simulink model "KalmanfilterReal"  (R2015a)
settings: Solver=ode3  StartTime=0.0  StopTime=10.0  FixedStep=1/200  RelTol=1e-3
undefined symbols (not defined in the file or in its folder): i
libraries: PoliArd x6
settings Model: ExtModeTrigDuration=2  Creator=User  LastModifiedBy=user
settings OptimizationCC: OptimizeModelRefInitCode=on  LifeSpan=1
settings DebuggingCC: UnderspecifiedInitializationDetection=Classic  MergeDetectMultiDrivingBlocksExec=none
settings HardwareCC: ProdLargestAtomicInteger=Long  ProdLargestAtomicFloat=Double  ProdEndianess=LittleEndian  ProdHWDeviceType=ARM Compatible->ARM Cortex
settings RTWCC: SystemTargetFile=realtime.tlc  GenerateMakefile=off  TemplateMakefile=realtime.tmf  Description=Run on Target Hardware  RTWVerbose=off
settings ERTTargetCC: CombineOutputUpdateFcns=off  ExtModeTransport=3  ExtModeMexFile=ext_serial_win32_comm_rtt  ExtModeMexArgs=0 1 9600  ERTSrcFileBannerTemplate=realtime_code_template.cgt  ERTHdrFileBannerTemplate=realtime_code_template.cgt  ERTDataSrcFileTemplate=realtime_code_template.cgt  ERTDataHdrFileTemplate=realtime_code_template.cgt  ERTCustomFileTemplate=realtime_file_process.tlc

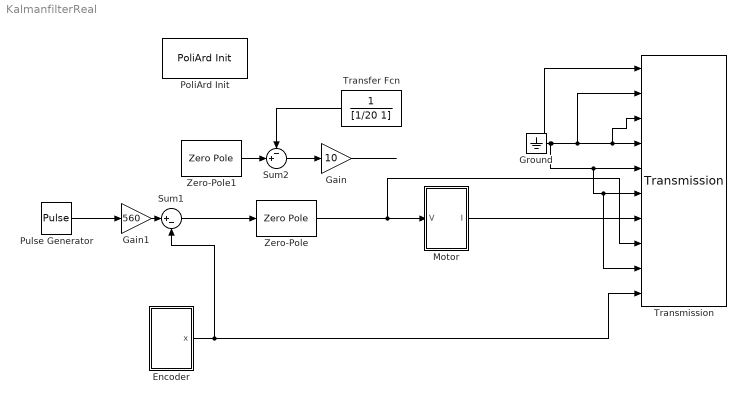
== system KalmanfilterReal ==
  "Encoder " : Subsystem
  Gain : Gain  Gain=10
  Gain1 : Gain  Gain=560
  Ground : Ground
  Motor : Subsystem
  PoliArd Init : PoliArd/PoliArd Init
  Pulse Generator : DiscretePulseGenerator  PulseType=Time based  Amplitude=-2.5  Period=10  PulseWidth=50  PhaseDelay=500
  Sum1 : Sum  Inputs=|+-
  Sum2 : Sum  Inputs=-+|
  Transfer Fcn : TransferFcn  Denominator=[1/20 1]
  Transmission : PoliArd/Transmission  sample_freq=200  sig_to_send=6
  Zero-Pole : ZeroPole  Zeros=[3.0405+i*12.6,3.0405-i*12.6]  Poles=[0 -200]  Gain=[-0.038702]
  Zero-Pole1 : ZeroPole  Zeros=[-2+22i, -2-22i]  Poles=[0, -100]  Gain=-0.1
  wires:
  Motor/1(I) -> Transmission/7
  Ground/1 -> Transmission/1, Transmission/9, Transmission/6, Transmission/5, Transmission/2, Transmission/3, Transmission/4
  Gain/1 -> ?
  Sum2/1 -> Gain/1
  Zero-Pole1/1 -> Sum2/2
  Transfer Fcn/1 -> Sum2/1
  Sum1/1 -> Zero-Pole/1
  Gain1/1 -> Sum1/1
  "Encoder "/1(x) -> Transmission/10, Sum1/2
  Zero-Pole/1 -> Transmission/8, Motor/1(V)
  Pulse Generator/1 -> Gain1/1

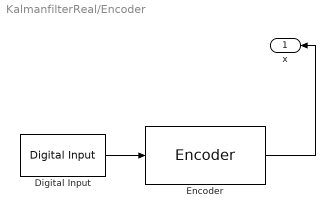
== system KalmanfilterReal/Encoder  ==
  Digital Input : PoliArd/Digital Input  DI_pin=2  DIsample=1/200
  Encoder : PoliArd/Encoder  EncoderID=1  dt_enc=-1
  x : Outport
  wires:
  Digital Input/1 -> Encoder/1
  Encoder/1 -> x/1

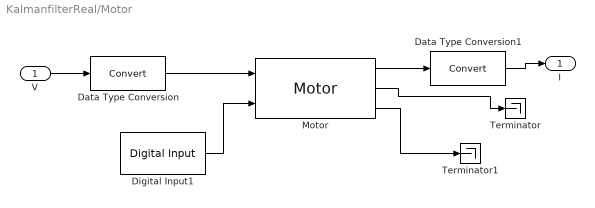
== system KalmanfilterReal/Motor ==
  V : Inport
  Data Type Conversion : DataTypeConversion
  Data Type Conversion1 : DataTypeConversion
  Digital Input1 : PoliArd/Digital Input  DI_pin=3  DIsample=1/200
  Motor : PoliArd/Motor  MotorID=1  DC_bus_mask=12  dt_mot=1/200
  Terminator : Terminator
  Terminator1 : Terminator
  I : Outport
  wires:
  Data Type Conversion/1 -> Motor/1
  Digital Input1/1 -> Motor/2
  V/1 -> Data Type Conversion/1
  Motor/3 -> Terminator1/1
  Motor/2 -> Terminator/1
  Motor/1 -> Data Type Conversion1/1
  Data Type Conversion1/1 -> I/1
